simulink model "relop_multi_test"  (Simulink 7.2)
settings: Solver=ode45  StartTime=0.0  StopTime=10.0  RelTol=1e-3
settings Model: Creator=arnaud  LastModifiedBy=arnaud
settings DataIOCC: SaveFormat=Structure

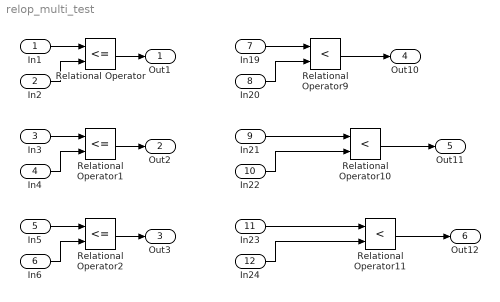
== system relop_multi_test ==
  In1 : Inport  PortDimensions=3  DataType=double  OutDataType=sfix(16)  OutScaling=2^0  OutDataTypeStr=double
  In2 : Inport  Port=2  PortDimensions=3  DataType=double  OutDataType=sfix(16)  OutScaling=2^0  OutDataTypeStr=double
  In3 : Inport  Port=3  PortDimensions=3  DataType=int8  OutDataType=sfix(16)  OutScaling=2^0  OutDataTypeStr=int8
  In4 : Inport  Port=4  PortDimensions=1  DataType=int8  OutDataType=sfix(16)  OutScaling=2^0  OutDataTypeStr=int8
  In5 : Inport  Port=5  PortDimensions=1  DataType=boolean  OutDataType=sfix(16)  OutScaling=2^0  OutDataTypeStr=boolean
  In6 : Inport  Port=6  PortDimensions=3  DataType=boolean  OutDataType=sfix(16)  OutScaling=2^0  OutDataTypeStr=boolean
  In19 : Inport  Port=7  PortDimensions=[2 3]  DataType=double  OutDataType=sfix(16)  OutScaling=2^0  OutDataTypeStr=double
  In20 : Inport  Port=8  PortDimensions=1  DataType=double  OutDataType=sfix(16)  OutScaling=2^0  OutDataTypeStr=double
  In21 : Inport  Port=9  PortDimensions=1  DataType=int8  OutDataType=sfix(16)  OutScaling=2^0  OutDataTypeStr=int8
  In22 : Inport  Port=10  PortDimensions=[2 3]  DataType=int8  OutDataType=sfix(16)  OutScaling=2^0  OutDataTypeStr=int8
  In23 : Inport  Port=11  PortDimensions=[2 3]  DataType=boolean  OutDataType=sfix(16)  OutScaling=2^0  OutDataTypeStr=boolean
  In24 : Inport  Port=12  PortDimensions=[2 3]  DataType=boolean  OutDataType=sfix(16)  OutScaling=2^0  OutDataTypeStr=boolean
  Relational Operator : RelationalOperator  Operator=<=  LogicOutDataTypeMode=boolean  OutDataTypeStr=boolean
  Relational Operator1 : RelationalOperator  Operator=<=  LogicOutDataTypeMode=boolean  OutDataTypeStr=boolean
  Relational Operator10 : RelationalOperator  Operator=<  LogicOutDataTypeMode=boolean  OutDataTypeStr=boolean
  Relational Operator11 : RelationalOperator  Operator=<  LogicOutDataTypeMode=boolean  OutDataTypeStr=boolean
  Relational Operator2 : RelationalOperator  Operator=<=  LogicOutDataTypeMode=boolean  OutDataTypeStr=boolean
  Relational Operator9 : RelationalOperator  Operator=<  LogicOutDataTypeMode=boolean  OutDataTypeStr=boolean
  Out1 : Outport  OutDataType=sfix(16)  OutScaling=2^0
  Out2 : Outport  Port=2  OutDataType=sfix(16)  OutScaling=2^0
  Out3 : Outport  Port=3  OutDataType=sfix(16)  OutScaling=2^0
  Out10 : Outport  Port=4  OutDataType=sfix(16)  OutScaling=2^0
  Out11 : Outport  Port=5  OutDataType=sfix(16)  OutScaling=2^0
  Out12 : Outport  Port=6  OutDataType=sfix(16)  OutScaling=2^0
  wires:
  In1/1 -> Relational Operator/1
  Relational Operator/1 -> Out1/1
  In2/1 -> Relational Operator/2
  In3/1 -> Relational Operator1/1
  Relational Operator1/1 -> Out2/1
  In4/1 -> Relational Operator1/2
  In5/1 -> Relational Operator2/1
  Relational Operator2/1 -> Out3/1
  In6/1 -> Relational Operator2/2
  In19/1 -> Relational Operator9/1
  Relational Operator9/1 -> Out10/1
  In20/1 -> Relational Operator9/2
  In21/1 -> Relational Operator10/1
  Relational Operator10/1 -> Out11/1
  In22/1 -> Relational Operator10/2
  In23/1 -> Relational Operator11/1
  Relational Operator11/1 -> Out12/1
  In24/1 -> Relational Operator11/2
